simulink model "model222b"  (R2024a)
settings: Solver=VariableStepAuto  StartTime=0.0  StopTime=10.0  RelTol=1e-3
settings Model: Creator=Xist  LastModifiedBy=Xist

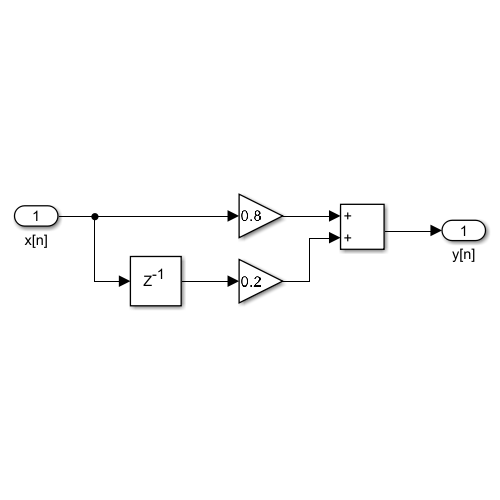
[thumbnail: Simulink's stored preview of the top-level diagram]
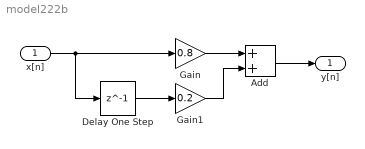
== system model222b ==
  x[n] : Inport
  Add : Sum
  Delay One Step : Delay  DelayLength=1
  Gain : Gain  Gain=0.8
  Gain1 : Gain  Gain=0.2
  y[n] : Outport
  wires:
  x[n]/1 -> Gain/1, Delay One Step/1
  Gain/1 -> Add/1
  Delay One Step/1 -> Gain1/1
  Gain1/1 -> Add/2
  Add/1 -> y[n]/1
